simulink model "PMC_bw"  (Simulink 7.0)
settings: Solver=ode4  SolverMode=SingleTasking  StartTime=0.0  StopTime=12  FixedStep=0.001  MaxStep=0.001  RelTol=1e-3  AbsTol=1e-3
undefined symbols (not defined in the file): mdlparamlist, pmcgain, pmctau2, pmctau3
CloseFcn:
  | ;slview('closediagram',bdroot);
settings Model: Creator=jacobs  LastModifiedBy=lfd  ExtModeAutoUpdateStatusClock=off
settings DataIOCC: LimitDataPoints=off  SaveOutput=off  SaveTime=off
settings OptimizationCC: BlockReduction=off  BooleanDataType=off
settings DebuggingCC: SaveWithParameterizedLinksMsg=none  SignalResolutionControl=TryResolveAllWithWarning  SolverPrmCheckMsg=none  MultiTaskDSMMsg=warning  MultiTaskCondExecSysMsg=none  StrictBusMsg=None
settings HardwareCC: TargetUnknown=on
settings RTWCC: IncludeERTFirstTime=on
settings GRTTargetCC: TargetFcnLib=ansi_tfl_tmw.mat  ModelReferenceCompliant=off  MatFileLogging=off

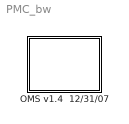
== system PMC_bw ==
  OMS v1.4  12/31/07 : Subsystem
      mask init:
      | k=0.25;loadmdlp;prolong_buffersize=5120;
      mask Display: disp('OMS v1.4\nModel')

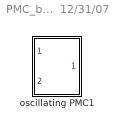
== system PMC_bw/OMS v1.4  12/31/07 ==
  oscillating PMC1 : Subsystem
      mask Display: disp('PMC+')

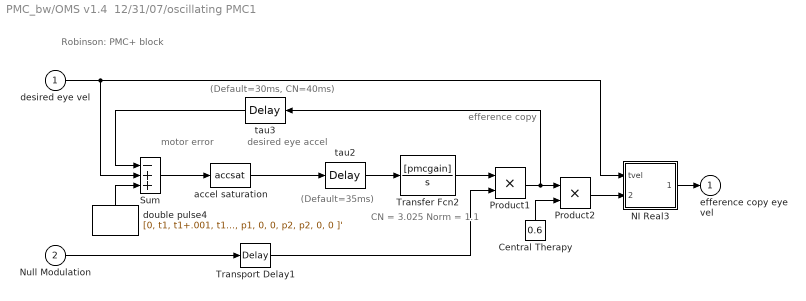
== system PMC_bw/OMS v1.4  12/31/07/oscillating PMC1 ==
  note: (Default=35ms)
  note: (Default=30ms, CN=40ms)
  note: CN = 3.025
      | Norm = 1.1
  note: efference
      | copy
  note: motor
      | error
  note: Robinson: PMC+ block
  note: desired
      | eye accel
  desired eye vel : Inport  OutDataType=sfix(16)  OutScaling=2^0
  Null Modulation : Inport  Port=2  OutDataType=sfix(16)  OutScaling=2^0
  Central Therapy : Constant  Orientation=up  Value=0.6  OutDataType=sfix(16)  OutScaling=2^0
  NI Real3 : Subsystem
      mask Display: disp('Velocity\nDeadzone')
  Product1 : Product  OutDataType=sfix(16)  OutScaling=2^0  SaturateOnIntegerOverflow=on  RndMeth=Zero  InputSameDT=on
  Product2 : Product  OutDataType=sfix(16)  OutScaling=2^0  SaturateOnIntegerOverflow=on  RndMeth=Zero  InputSameDT=on
  Sum : Sum  Inputs=-++  OutDataType=sfix(16)  OutScaling=2^0  SaturateOnIntegerOverflow=on  InputSameDT=on
  Transfer Fcn2 : TransferFcn  Numerator=[pmcgain]  Denominator=[1 0]
  Transport Delay1 : TransportDelay  DelayTime=0.025
      mask Display: disp('25ms')
  accel saturation : MATLABFcn  MATLABFcn=accsat
      mask Display: plot([-80 -4 4 80],[-120 -40 40 120], [0 0],[-120 120],[-80 80],[0 0])
  double pulse4 : FromWorkspace  Orientation=up  VariableName=[0, t1, t1+.001, t1+d1, t1+d1+.001, t1+d1+.001+ipd, t1+d1+.001+ipd, t1+d1+.001+ipd+d2, t1+d1+.001+ipd+d2, 10000; 0, 0, p1, p1, 0, 0, p2, p2, 0, 0 ]'  SampleTime=.001  mask{@1=825, @2=0, @3=.002, @4=.050, @5=-925, @6=.002}
      mask prompts: @1 "Pulse 1 Magnitude"; @2 "Time of Pulse 1 Onset"; @3 "Pulse 1 Duration"; @4 "Interpulse Delay"; @5 "Pulse 2 Magnitude"; @6 "Pulse 2 Duration"
      mask help: Double Pulse
      mask init:
      | p1=@1; t1=@2; d1=@3; ipd=@4; p2=@5; d2=@6;
      mask Display: disp('Double\nPulse')
  tau2 : TransportDelay  DelayTime=pmctau2/1000
  tau3 : TransportDelay  Orientation=left  DelayTime=pmctau3/1000
  efference copy eye vel : Outport  OutDataType=sfix(16)  OutScaling=2^0  InitialOutput=0
  wires:
  Central Therapy/1 -> Product2/2
  Product2/1 -> NI Real3/2(ecpyvel)
  NI Real3/1(ecpyveldz) -> efference copy eye vel/1
  Product1/1 -> Product2/1, tau3/1
  Null Modulation/1 -> Transport Delay1/1
  double pulse4/1 -> Sum/3
  desired eye vel/1 -> NI Real3/1(tvel), Sum/2
  tau3/1 -> Sum/1
  Sum/1 -> accel saturation/1
  tau2/1 -> Transfer Fcn2/1
  accel saturation/1 -> tau2/1
  Transfer Fcn2/1 -> Product1/1
  Transport Delay1/1 -> Product1/2

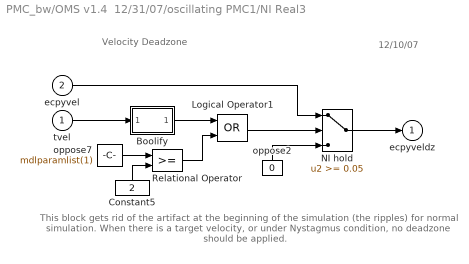
== system PMC_bw/OMS v1.4  12/31/07/oscillating PMC1/NI Real3 ==
  note: This block gets rid of the artifact at the beginning of the simulation
      | (the ripples) for normal simulation.
      | When there is a target velocity, or under Nystagmus condition, no deadzone should be applied.
  note: 12/10/07
  note: Velocity Deadzone
  tvel : Inport  OutDataType=sfix(16)  OutScaling=2^0
  ecpyvel : Inport  Port=2  OutDataType=sfix(16)  OutScaling=2^0
  Boolify : Subsystem
      mask Display: disp('Boolify')
  Constant5 : Constant  Orientation=up  Value=2  OutDataType=sfix(16)  OutScaling=2^0
  Logical Operator1 : Logic  Operator=OR
  NI hold : Switch  Threshold=0.05  SaturateOnIntegerOverflow=on  InputSameDT=on
  Relational Operator : RelationalOperator  InputSameDT=on
  oppose2 : Constant  Orientation=up  Value=0  OutDataType=sfix(16)  OutScaling=2^0
  oppose7 : Constant  Value=mdlparamlist(1)  OutDataType=sfix(16)  OutScaling=2^0
  ecpyveldz : Outport  OutDataType=sfix(16)  OutScaling=2^0  InitialOutput=0
  wires:
  NI hold/1 -> ecpyveldz/1
  ecpyvel/1 -> NI hold/1
  oppose2/1 -> NI hold/3
  Logical Operator1/1 -> NI hold/2
  Relational Operator/1 -> Logical Operator1/2
  oppose7/1 -> Relational Operator/1
  Constant5/1 -> Relational Operator/2
  Boolify/1(Out1) -> Logical Operator1/1
  tvel/1 -> Boolify/1(In1)

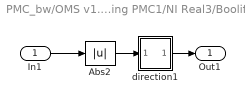
== system PMC_bw/OMS v1.4  12/31/07/oscillating PMC1/NI Real3/Boolify ==
  In1 : Inport  OutDataType=sfix(16)  OutScaling=2^0
  Abs2 : Abs  SaturateOnIntegerOverflow=on
  direction1 : Subsystem
      mask Type: Sign
      mask Description: y = sign(x)
      mask Help: Sign Function:\n\t\t\ty = 1 if x > 0\n\t\t\ty = 0 if x = 0\n\t\t\ty = -1 if x < 0
      mask Display: plot(-50,-50,50,50,[-50,50],[0,0],[0,0],[-50,50],[-40,0],[-30,-30],[0,40],[30,30])
  Out1 : Outport  OutDataType=sfix(16)  OutScaling=2^0  InitialOutput=0
  wires:
  direction1/1(out_1) -> Out1/1
  In1/1 -> Abs2/1
  Abs2/1 -> direction1/1(in_1)

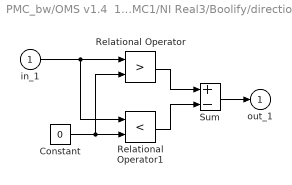
== system PMC_bw/OMS v1.4  12/31/07/oscillating PMC1/NI Real3/Boolify/direction1 ==
  in_1 : Inport  OutDataType=sfix(16)  OutScaling=2^0
  Constant : Constant  Value=0  OutDataType=sfix(16)  OutScaling=2^0
  Relational Operator : RelationalOperator  Operator=>  InputSameDT=on
  Relational Operator1 : RelationalOperator  Operator=<  InputSameDT=on
  Sum : Sum  Inputs=+-  OutDataType=sfix(16)  OutScaling=2^0  SaturateOnIntegerOverflow=on  InputSameDT=on
  out_1 : Outport  OutDataType=sfix(16)  OutScaling=2^0  InitialOutput=0
  wires:
  Sum/1 -> out_1/1
  Relational Operator/1 -> Sum/1
  Relational Operator1/1 -> Sum/2
  Constant/1 -> Relational Operator/2, Relational Operator1/2
  in_1/1 -> Relational Operator1/1, Relational Operator/1
